simulink model "cfd_pulse_shaping"  (R2020b)
settings: Solver=VariableStepAuto  StartTime=0.0  StopTime=4.1e-6  RelTol=1e-3
values from neighbouring files (symbols this model uses):
  nakhostin_10_1_eneg = exp(-sampling_rate/2/hpf_diff_constant)    [file_pulse_shaping_params.m]    (also in pulse_shaping_params.m)
  nakhostin_10_1_epos = exp(sampling_rate/2/hpf_diff_constant)    [file_pulse_shaping_params.m]    (also in pulse_shaping_params.m)
  nakhostin_10_1_v0 = 2^15    (= 32768)    [file_pulse_shaping_params.m]
  sampling_period = 1e-9    (= 1e-09)    [ascii_to_mat.m]    (also in file_pulse_shaping_params.m; symbolic_biexponential.m)
libraries: dspstat3 x1
settings Model: Creator=Dickbutt  LastModifiedBy=Dickbutt

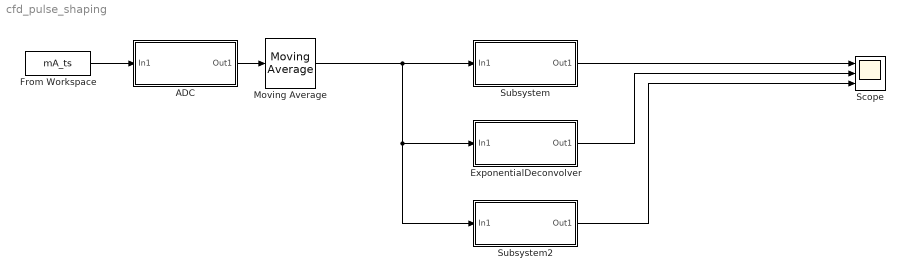
== system cfd_pulse_shaping ==
  ADC : Subsystem
  ExponentialDeconvolver : Subsystem
  From Workspace : FromWorkspace  VariableName=mA_ts  SampleTime=sampling_period  Interpolate=off  ZeroCross=off  OutputAfterFinalValue=Setting to zero
  Moving Average : dspstat3/Moving Average  Method=Sliding window  ForgettingFactorPort=off  SpecifyWindowLength=on  WindowLength=primary_ma  ForgettingFactor=0.9  SimulateUsing=Code generation
  Scope : Scope  NumInputPorts=3
  Subsystem : Subsystem
  Subsystem2 : Subsystem
  wires:
  From Workspace/1 -> ADC/1(In1)
  ADC/1(Out1) -> Moving Average/1
  Moving Average/1 -> Subsystem2/1(In1), ExponentialDeconvolver/1(In1), Subsystem/1(In1)
  Subsystem/1(Out1) -> Scope/1
  ExponentialDeconvolver/1(Out1) -> Scope/2
  Subsystem2/1(Out1) -> Scope/3

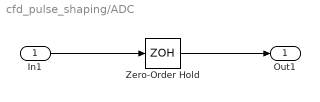
== system cfd_pulse_shaping/ADC ==
  In1 : Inport
  Zero-Order Hold : ZeroOrderHold  SampleTime=sampling_period
  Out1 : Outport
  wires:
  In1/1 -> Zero-Order Hold/1
  Zero-Order Hold/1 -> Out1/1

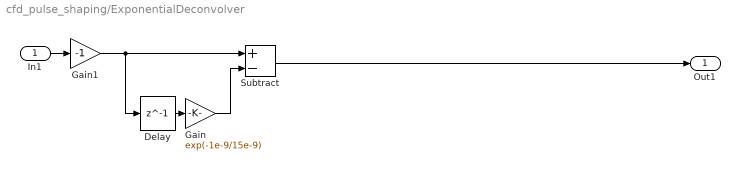
== system cfd_pulse_shaping/ExponentialDeconvolver ==
  In1 : Inport
  Delay : Delay  DelayLength=1  InitialCondition=0
  Gain : Gain  Gain=exp(-1e-9/15e-9)
  Gain1 : Gain  Gain=-1
  Subtract : Sum  Inputs=+-
  Out1 : Outport
  wires:
  In1/1 -> Gain1/1
  Gain1/1 -> Delay/1, Subtract/1
  Subtract/1 -> Out1/1
  Delay/1 -> Gain/1
  Gain/1 -> Subtract/2

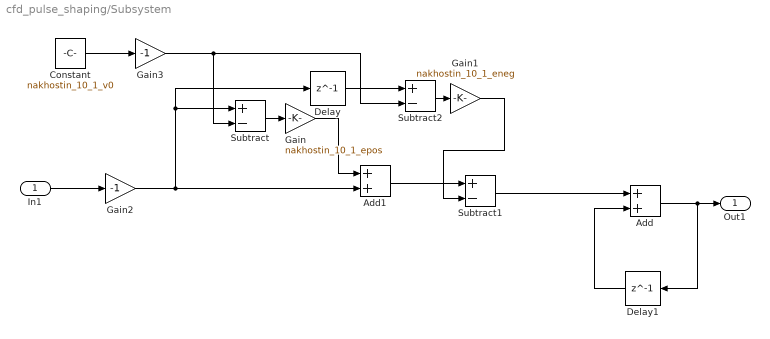
== system cfd_pulse_shaping/Subsystem ==
  In1 : Inport
  Add : Sum
  Add1 : Sum
  Constant : Constant  Value=nakhostin_10_1_v0
  Delay : Delay  DelayLength=1  InitialCondition=0
  Delay1 : Delay  DelayLength=1  InitialCondition=0
  Gain : Gain  Gain=nakhostin_10_1_epos
  Gain1 : Gain  Gain=nakhostin_10_1_eneg
  Gain2 : Gain  Gain=-1
  Gain3 : Gain  Gain=-1
  Subtract : Sum  Inputs=+-
  Subtract1 : Sum  Inputs=+-
  Subtract2 : Sum  Inputs=+-
  Out1 : Outport
  wires:
  In1/1 -> Gain2/1
  Delay1/1 -> Add/2
  Constant/1 -> Gain3/1
  Add/1 -> Delay1/1, Out1/1
  Subtract/1 -> Gain/1
  Gain/1 -> Add1/1
  Add1/1 -> Subtract1/1
  Subtract2/1 -> Gain1/1
  Gain1/1 -> Subtract1/2
  Delay/1 -> Subtract2/1
  Subtract1/1 -> Add/1
  Gain2/1 -> Delay/1, Subtract/1, Add1/2
  Gain3/1 -> Subtract/2, Subtract2/2

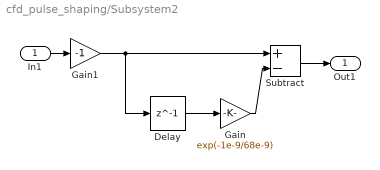
== system cfd_pulse_shaping/Subsystem2 ==
  In1 : Inport
  Delay : Delay  DelayLength=1  InitialCondition=0
  Gain : Gain  Gain=exp(-1e-9/68e-9)
  Gain1 : Gain  Gain=-1
  Subtract : Sum  Inputs=+-
  Out1 : Outport
  wires:
  In1/1 -> Gain1/1
  Gain1/1 -> Delay/1, Subtract/1
  Subtract/1 -> Out1/1
  Delay/1 -> Gain/1
  Gain/1 -> Subtract/2
